simulink model "FcDegRecSubModel_01"  (R2022b)
settings: Solver=VariableStepAuto  StartTime=0.0  StopTime=max(Driving_cycle_v_kmph(:,1))  RelTol=1e-3
undefined symbols (not defined in the file or in its folder): usd2rmb
settings Model: Creator=xuupp  LastModifiedBy=xuupp

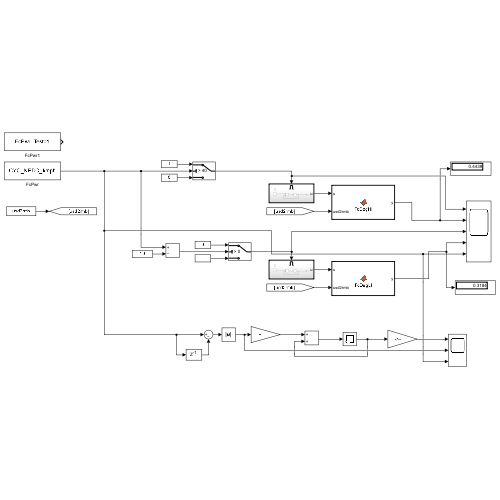
[thumbnail: Simulink's stored preview of the top-level diagram]
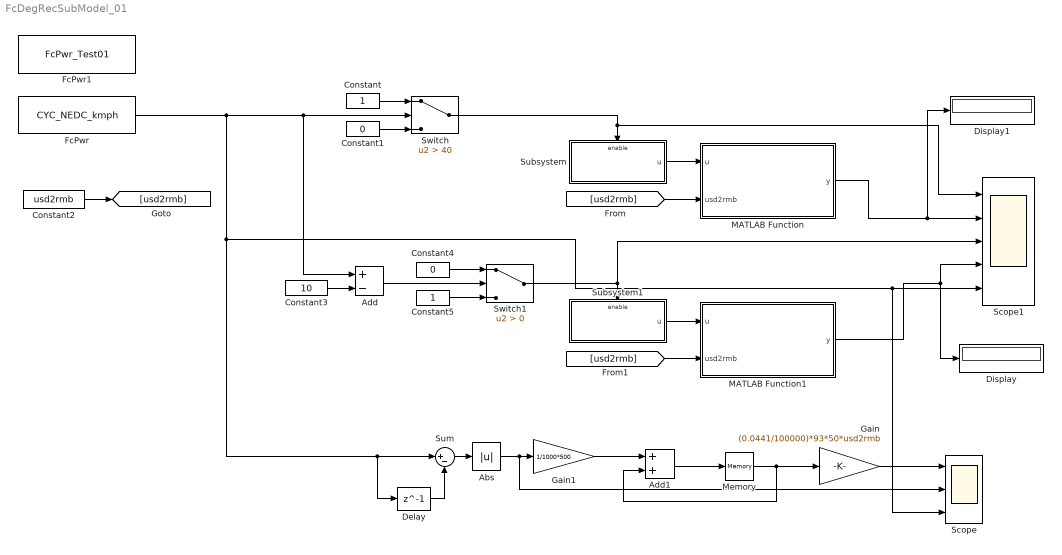
== system FcDegRecSubModel_01 ==
  Abs : Abs  SaturateOnIntegerOverflow=off
  Add : Sum  Inputs=+-
  Add1 : Sum
  Constant : Constant
  Constant1 : Constant  Value=0
  Constant2 : Constant  Value=usd2rmb
  Constant3 : Constant  Value=10
  Constant4 : Constant  Value=0
  Constant5 : Constant
  Delay : Delay  DelayLength=1
  Display : Display
  Display1 : Display
  FcPwr : FromWorkspace  VariableName=CYC_NEDC_kmph  SampleTime=1  ZeroCross=off
  FcPwr1 : FromWorkspace  VariableName=FcPwr_Test01  SampleTime=1  ZeroCross=off
  Gain : Gain  Gain=(0.0441/100000)*93*50*usd2rmb
  Gain1 : Gain  Gain=1/1000*500
  MATLAB Function : MATLAB Function  TreatAsAtomicUnit=on
  MATLAB Function1 : MATLAB Function  TreatAsAtomicUnit=on
  Memory : Memory
  Scope : Scope  NumInputPorts=3
  Scope1 : Scope  NumInputPorts=5
  Subsystem : Subsystem
  Subsystem1 : Subsystem
  Sum : Sum  Inputs=|+-
  Switch : Switch  Criteria=u2 > Threshold  Threshold=40  SaturateOnIntegerOverflow=off  InputSameDT=off
  Switch1 : Switch  Criteria=u2 > Threshold  SaturateOnIntegerOverflow=off  InputSameDT=off
  wires:
  FcPwr/1 -> Scope/3, Scope1/5, Sum/1, Delay/1, Add/1, Switch/2
  Constant/1 -> Switch/1
  Constant1/1 -> Switch/3
  Switch/1 -> Subsystem/Enable, Scope1/1
  Subsystem/1(u) -> MATLAB Function/1(u)
  [usd2rmb] -> MATLAB Function/2(usd2rmb)
  Subsystem1/1(u) -> MATLAB Function1/1(u)
  [usd2rmb] -> MATLAB Function1/2(usd2rmb)
  Constant3/1 -> Add/2
  Add/1 -> Switch1/2
  Constant4/1 -> Switch1/1
  Constant5/1 -> Switch1/3
  Switch1/1 -> Subsystem1/Enable, Scope1/3
  MATLAB Function/1(y) -> Display1/1, Scope1/2
  MATLAB Function1/1(y) -> Display/1, Scope1/4
  Delay/1 -> Sum/2
  Sum/1 -> Abs/1
  Abs/1 -> Scope/2, Gain1/1
  Add1/1 -> Memory/1
  Memory/1 -> Gain/1, Add1/2
  Gain1/1 -> Add1/1
  Constant2/1 -> [usd2rmb]
  Gain/1 -> Scope/1

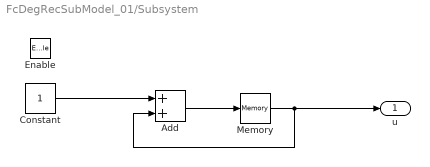
== system FcDegRecSubModel_01/Subsystem ==
  Enable : EnablePort
  Add : Sum
  Constant : Constant
  Memory : Memory
  u : Outport
  wires:
  Constant/1 -> Add/1
  Add/1 -> Memory/1
  Memory/1 -> Add/2, u/1

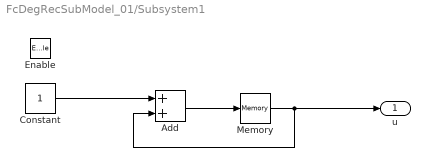
== system FcDegRecSubModel_01/Subsystem1 ==
  Enable : EnablePort
  Add : Sum
  Constant : Constant
  Memory : Memory
  u : Outport
  wires:
  Memory/1 -> u/1, Add/2
  Add/1 -> Memory/1
  Constant/1 -> Add/1

== matlab function FcDegRecSubModel_01/MATLAB Function ==
  data: u input; y output; usd2rmb input
function y = FcDegHl(u,usd2rmb)
alpha_h = 10;   %10e-6V/h
u_eol = 100000;   %10e-6V
p_stack = 50*93*usd2rmb;

y = (alpha_h*p_stack/u_eol)*u/3600;

== matlab function FcDegRecSubModel_01/MATLAB Function1 ==
  data: u input; y output; usd2rmb input
function y = FcDegLl(u,usd2rmb)
alpha_l = 8.66;   %10e-6V/h
u_eol = 100000;   %10e-6V
p_stack = 50*93*usd2rmb;

y = (alpha_l*p_stack/u_eol)*u/3600;
